simulink model "TailSitter_Sim"  (R2025b)
settings: Solver=ode3  StartTime=0.0  StopTime=10.0  FixedStep=0.01  RelTol=1e-3  EnableMultiTasking=on
values from neighbouring files (symbols this model uses):
  Ixx = 0.005    [Init.m]
  Iyy = 0.005    [Init.m]
  Izz = 0.009    [Init.m]
  m = 0.5    [Init.m]
  M_alloc = [  c_T,     c_T,     c_T,     c_T ... (first row only)    [Init.m]
  max_rpm = KV *Ub    (= 15540)    [Init.m]
settings Model: Creator=Murat  LastModifiedBy=Murat
settings OptimizationCC: DefaultParameterBehavior=Inlined  EnhancedBackFolding=on  PassReuseOutputArgsAs=Individual arguments  ZeroExternalMemoryAtStartup=off  ZeroInternalMemoryAtStartup=off  MaxStackSize=64  OptimizeBlockOrder=speed  DifferentSizesBufferReuse=on  OptimizationCustomize=off  EfficientTunableParamExpr=on
settings DebuggingCC: ParameterTunabilityLossMsg=error
settings HardwareCC: ProdBitPerPointer=32.0  ProdBitPerSizeT=32.0  ProdBitPerPtrDiffT=32.0  ProdLargestAtomicInteger=Long  ProdLargestAtomicFloat=Double  ProdWordSize=32.0  ProdLongLongMode=on  ProdHWDeviceType=ARM Compatible->ARM Cortex-M
settings SFSimCC: MATLABDynamicMemAlloc=off
settings RTWCC: SystemTargetFile=ert.tlc  PackageGeneratedCodeAndArtifacts=on  TemplateMakefile=ert_default_tmf  Toolchain=GNU Tools for ARM Embedded Processors  BuildConfiguration=Specify  Description=Embedded Coder
settings CodeAppCC: ForceParamTrailComments=on  IgnoreCustomStorageClasses=off  OperatorAnnotations=on  SimulinkDataObjDesc=on  SFDataObjDesc=on  InsertBlockDesc=on
settings ERTTargetCC: ExtModeTransport=3.0  ExtModeStaticAlloc=on  ExtModeStaticAllocSize=2048.0  ExtModeMexFile=ext_xcp  ExtModeIntrfLevel=Level2 - Open  ERTCustomFileTemplate=example_file_process.tlc  TargetLangStandard=C99 (ISO)  CodeReplacementLibrary=ARM Cortex-M  SupportContinuousTime=on

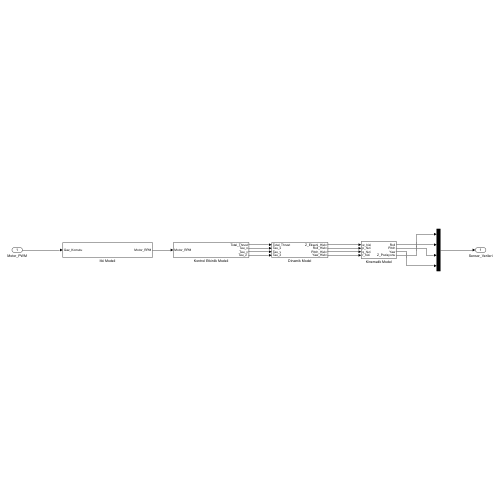
[thumbnail: Simulink's stored preview of the top-level diagram]
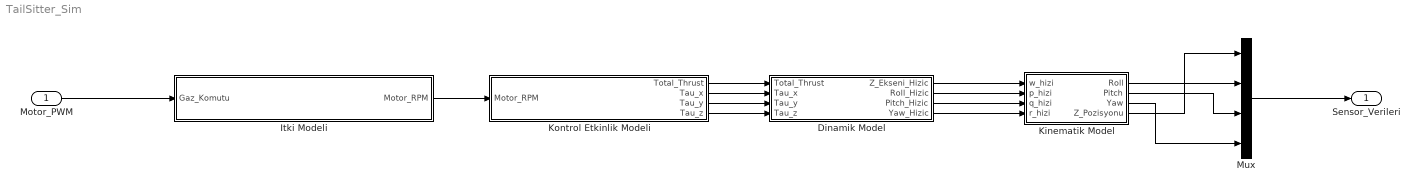
== system TailSitter_Sim ==
  Motor_PWM : Inport
  Dinamik Model : Subsystem
  Itki Modeli : Subsystem
  Kinematik Model : Subsystem
  Kontrol Etkinlik Modeli : Subsystem
  Mux : Mux
  Sensor_Verileri : Outport
  wires:
  Itki Modeli/1(Motor_RPM) -> Kontrol Etkinlik Modeli/1(Motor_RPM)
  Kontrol Etkinlik Modeli/1(Total_Thrust) -> Dinamik Model/1(Total_Thrust)
  Kontrol Etkinlik Modeli/2(Tau_x) -> Dinamik Model/2(Tau_x)
  Kontrol Etkinlik Modeli/3(Tau_y) -> Dinamik Model/3(Tau_y)
  Kontrol Etkinlik Modeli/4("Tau_z ") -> Dinamik Model/4(Tau_z)
  Dinamik Model/1(Z_Ekseni_Hizic) -> Kinematik Model/1(w_hizi)
  Dinamik Model/2(Roll_Hizic) -> Kinematik Model/2(p_hizi)
  Dinamik Model/3(Pitch_Hizic) -> Kinematik Model/3("q_hizi ")
  Dinamik Model/4(Yaw_Hizic) -> Kinematik Model/4("r_hizi ")
  Kinematik Model/4(Z_Pozisyonu) -> Mux/1
  Kinematik Model/1(Roll) -> Mux/2
  Kinematik Model/2(Pitch) -> Mux/3
  Kinematik Model/3(Yaw) -> Mux/4
  Motor_PWM/1 -> Itki Modeli/1(Gaz_Komutu)
  Mux/1 -> Sensor_Verileri/1

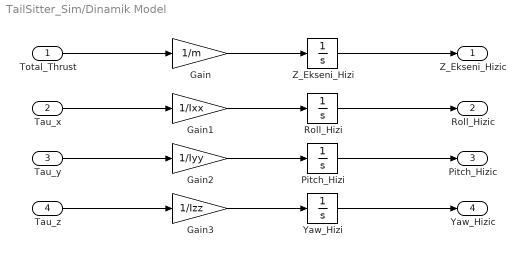
== system TailSitter_Sim/Dinamik Model ==
  Total_Thrust : Inport
  Tau_x : Inport  Port=2
  Tau_y : Inport  Port=3
  Tau_z : Inport  Port=4
  " Pitch_Hizi" : Integrator
  Gain : Gain  Gain=1/m
  Gain1 : Gain  Gain=1/Ixx
  Gain2 : Gain  Gain=1/Iyy
  Gain3 : Gain  Gain=1/Izz
  "Roll_Hizi " : Integrator
  "Yaw_Hizi " : Integrator
  Z_Ekseni_Hizi : Integrator
  Z_Ekseni_Hizic : Outport
  Roll_Hizic : Outport  Port=2
  Pitch_Hizic : Outport  Port=3
  Yaw_Hizic : Outport  Port=4
  wires:
  Total_Thrust/1 -> Gain/1
  Tau_x/1 -> Gain1/1
  Tau_y/1 -> Gain2/1
  Tau_z/1 -> Gain3/1
  Gain/1 -> Z_Ekseni_Hizi/1
  Gain1/1 -> "Roll_Hizi "/1
  Gain2/1 -> " Pitch_Hizi"/1
  Gain3/1 -> "Yaw_Hizi "/1
  Z_Ekseni_Hizi/1 -> Z_Ekseni_Hizic/1
  "Roll_Hizi "/1 -> Roll_Hizic/1
  " Pitch_Hizi"/1 -> Pitch_Hizic/1
  "Yaw_Hizi "/1 -> Yaw_Hizic/1

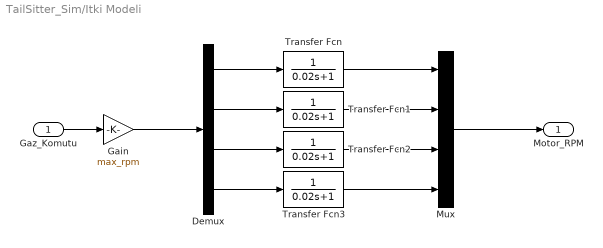
== system TailSitter_Sim/Itki Modeli ==
  Gaz_Komutu : Inport
  Demux : Demux
  Gain : Gain  Gain=max_rpm
  Mux : Mux
  Transfer Fcn{,1..3} (4 alike) : TransferFcn  Denominator=[0.02 1]
  Motor_RPM : Outport
  wires:
  Gaz_Komutu/1 -> Gain/1
  Gain/1 -> Demux/1
  Demux/1 -> Transfer Fcn/1
  Demux/2 -> Transfer Fcn1/1
  Demux/3 -> Transfer Fcn2/1
  Demux/4 -> Transfer Fcn3/1
  Transfer Fcn/1 -> Mux/1
  Transfer Fcn1/1 -> Mux/2
  Transfer Fcn2/1 -> Mux/3
  Transfer Fcn3/1 -> Mux/4
  Mux/1 -> Motor_RPM/1

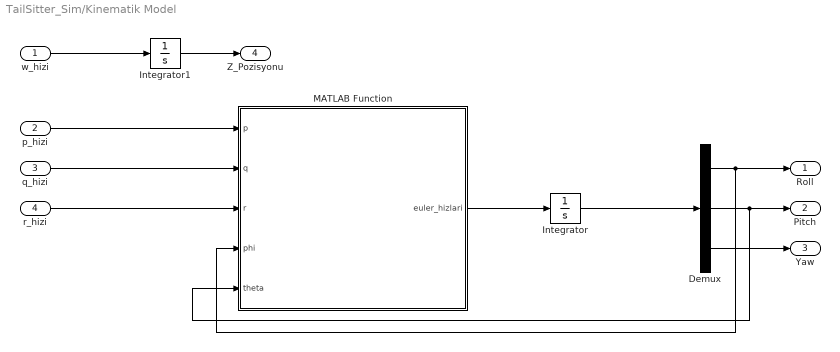
== system TailSitter_Sim/Kinematik Model ==
  w_hizi : Inport
  p_hizi : Inport  Port=2
  "q_hizi " : Inport  Port=3
  "r_hizi " : Inport  Port=4
  Demux : Demux  Outputs=3
  Integrator : Integrator
  Integrator1 : Integrator
  MATLAB Function : MATLAB Function  TreatAsAtomicUnit=on
  Roll : Outport
  Pitch : Outport  Port=2
  Yaw : Outport  Port=3
  Z_Pozisyonu : Outport  Port=4
  wires:
  p_hizi/1 -> MATLAB Function/1(p)
  "q_hizi "/1 -> MATLAB Function/2(q)
  "r_hizi "/1 -> MATLAB Function/3(r)
  MATLAB Function/1(euler_hizlari) -> Integrator/1
  Integrator/1 -> Demux/1
  Demux/1 -> MATLAB Function/4(phi), Roll/1
  Demux/2 -> MATLAB Function/5(theta), Pitch/1
  Demux/3 -> Yaw/1
  w_hizi/1 -> Integrator1/1
  Integrator1/1 -> Z_Pozisyonu/1

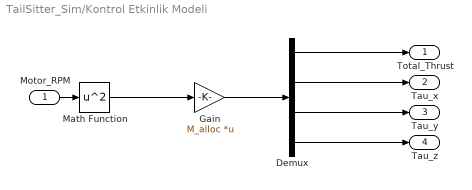
== system TailSitter_Sim/Kontrol Etkinlik Modeli ==
  Motor_RPM : Inport
  Demux : Demux
  Gain : Gain  Gain=M_alloc  Multiplication=Matrix(K*u)
  Math Function : Math  Operator=square
  Total_Thrust : Outport
  Tau_x : Outport  Port=2
  Tau_y : Outport  Port=3
  "Tau_z " : Outport  Port=4
  wires:
  Motor_RPM/1 -> Math Function/1
  Math Function/1 -> Gain/1
  Gain/1 -> Demux/1
  Demux/1 -> Total_Thrust/1
  Demux/2 -> Tau_x/1
  Demux/3 -> Tau_y/1
  Demux/4 -> "Tau_z "/1

== matlab function TailSitter_Sim/Kinematik Model/MATLAB Function ==
  data: p input; euler_hizlari output; q input; r input; phi input; theta input
function euler_hizlari = euler_kinematik(p, q, r, phi, theta)
    % Euler Kinematik Donusum Matrisi
    R = [1, sin(phi)*tan(theta), cos(phi)*tan(theta);
         0, cos(phi),            -sin(phi);
         0, sin(phi)/cos(theta), cos(phi)/cos(theta)];
         
    euler_hizlari = R * [p; q; r];
end
